simulink model "without_pid"  (R2014a)
settings: Solver=ode45  StartTime=0.0  StopTime=10.0  RelTol=1e-3
libraries: simulink x1
settings Model: Creator=gmerritt  LastModifiedBy=gmerritt

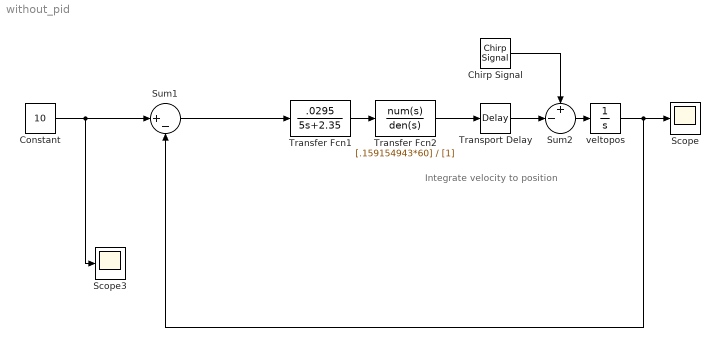
== system without_pid ==
  note: Integrate velocity to position
  Chirp Signal : simulink/Sources/Chirp Signal  f1=0.1  T=100  f2=.8
  Constant : Constant  Value=10
  Scope : Scope
      settings: SaveName=output
  Scope3 : Scope
      settings: SaveName=input1
  Sum1 : Sum  Inputs=|+-
  Sum2 : Sum  Inputs=+-|
  Transfer Fcn1 : TransferFcn  Numerator=[.0295]  Denominator=[5 2.35]
  Transfer Fcn2 : TransferFcn  Numerator=[.159154943*60]  Denominator=[1]
  Transport Delay : TransportDelay
  "veltopos " : Integrator
  wires:
  Transfer Fcn1/1 -> Transfer Fcn2/1
  Transfer Fcn2/1 -> Transport Delay/1
  Sum2/1 -> "veltopos "/1
  Transport Delay/1 -> Sum2/2
  Sum1/1 -> Transfer Fcn1/1
  "veltopos "/1 -> Sum1/2, Scope/1
  Constant/1 -> Scope3/1, Sum1/1
  Chirp Signal/1 -> Sum2/1
